simulink model "ABS_Quadrotor"  (R2017b)
settings: Solver=VariableStepAuto  StartTime=0.0  StopTime=10.0  RelTol=1e-3
undefined symbols (not defined in the file): ct, dctcq, quad
libraries: shared6dof x1
settings Model: Creator=hoang  LastModifiedBy=hoang

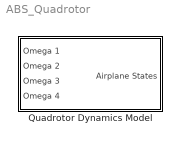
== system ABS_Quadrotor ==
  Quadrotor Dynamics Model : Subsystem

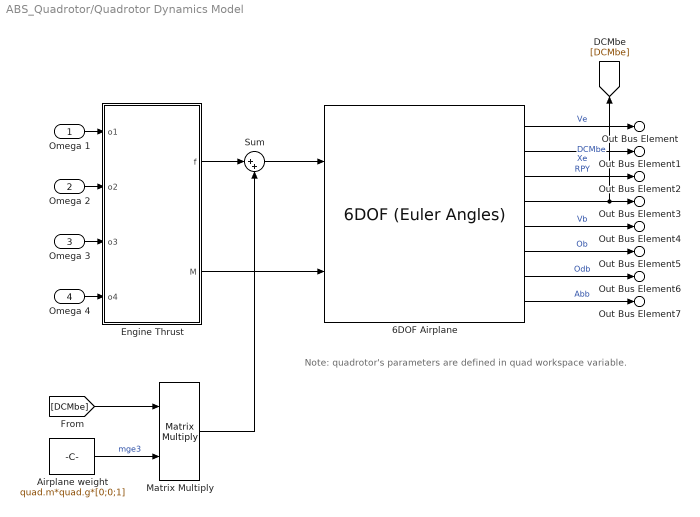
== system ABS_Quadrotor/Quadrotor Dynamics Model ==
  note: Note: quadrotor's parameters are defined in quad workspace variable.
  Omega 1 : Inport
  Omega 2 : Inport  Port=2
  Omega 3 : Inport  Port=3
  Omega 4 : Inport  Port=4
  6DOF Airplane : shared6dof/6DOF (Euler Angles)  units=Metric (MKS)  mtype=Fixed  rep=Euler Angles  xme_0=[0 0 0]  Vm_0=[0 0 0]  eul_0=[0 0 0]  pm_0=[0 0 0]  mass_0=quad.m  mass_e=0.5  mass_f=2.0  inertia=quad.J  inertia_e=eye(3)  inertia_f=2*eye(3)  k_quat=1.0  vre_flag=on  abi_flag=off
      settings: SourceProductBaseCode=AE
  Airplane weight : Constant  Value=quad.m*quad.g*[0;0;1]
  Engine Thrust : MATLAB Function  TreatAsAtomicUnit=on
  Matrix Multiply : Product  Multiplication=Matrix(*)
  Sum : Sum  Inputs=|++
  Out Bus Element : Outport  PortName=Airplane States  Element=Ve
  Out Bus Element1 : Outport  PortName=Airplane States  Element=Xe
  Out Bus Element2 : Outport  PortName=Airplane States  Element=RPY
  Out Bus Element3 : Outport  PortName=Airplane States  Element=DCMbe
  Out Bus Element4 : Outport  PortName=Airplane States  Element=Vb
  Out Bus Element5 : Outport  PortName=Airplane States  Element=Ob
  Out Bus Element6 : Outport  PortName=Airplane States  Element=Odb
  Out Bus Element7 : Outport  PortName=Airplane States  Element=Abb
  wires:
  6DOF Airplane/6 -> Out Bus Element5/1  "Ob"
  Airplane weight/1 -> Matrix Multiply/2  "mge3"
  Engine Thrust/1(f) -> Sum/1
  Matrix Multiply/1 -> Sum/2
  6DOF Airplane/1 -> Out Bus Element/1  "Ve"
  6DOF Airplane/3 -> Out Bus Element2/1  "RPY"
  6DOF Airplane/4 -> Out Bus Element3/1, [DCMbe]  "DCMbe"
  6DOF Airplane/2 -> Out Bus Element1/1  "Xe"
  6DOF Airplane/7 -> Out Bus Element6/1  "Odb"
  6DOF Airplane/5 -> Out Bus Element4/1  "Vb"
  6DOF Airplane/8 -> Out Bus Element7/1  "Abb"
  Engine Thrust/2(M) -> 6DOF Airplane/2
  Sum/1 -> 6DOF Airplane/1
  Omega 2/1 -> Engine Thrust/2(o2)
  Omega 3/1 -> Engine Thrust/3(o3)
  Omega 4/1 -> Engine Thrust/4(o4)
  Omega 1/1 -> Engine Thrust/1(o1)
  [DCMbe] -> Matrix Multiply/1

== matlab function ABS_Quadrotor/Quadrotor Dynamics Model/Engine Thrust ==
  data: o1 input size=1; f output size=[3 1]; o2 input size=1; o3 input size=1; o4 input size=1; M output size=[3 1]; ct parameter; dctcq parameter size=[3 4]
function [f,M] = fcn(o1,o2,o3,o4,ct, dctcq)
[f,M] = omega2force(o1,o2,o3,o4,ct,dctcq);
